simulink model "analysis_PI_ctrl_lin_uncertain_model_z"  (R2020b)
settings: Solver=FixedStepAuto  StartTime=0.0  StopTime=10.0  FixedStep=1e-3  RelTol=1e-3
values from neighbouring files (symbols this model uses):
  B = 10    [hinfCostFunc.m]    (also in hinf_analysis_z.m; hinf_cmd_lmi.m = [zeros(4,2); Sigma.B]; init_rob_synth_sim.m; muCostFunc.m = 11)
  dq0 = [0;0;0]    [hinfCostFunc.m]    (also in hinf_analysis_z.m; init_rob_synth_sim.m = [0; 0; 0]; muCostFunc.m; mu_analysis_z.m)
  Ki = 0.08    [hinfCostFunc.m]    (also in hinf_analysis_z.m; muCostFunc.m; mu_analysis_z.m; robust_synthesis.m)
  Kp = 0.015    [hinfCostFunc.m]    (also in hinf_analysis_z.m; muCostFunc.m; mu_analysis_z.m; robust_synthesis.m)
  M = 0.45    [hinfCostFunc.m]    (also in hinf_analysis_z.m; init_rob_synth_sim.m; muCostFunc.m = 0.42; mu_analysis_z.m = 0.42)
  q0 = [1.676; -4.363; 1.497]    [hinfCostFunc.m]    (also in hinf_analysis_z.m; init_rob_synth_sim.m; muCostFunc.m; mu_analysis_z.m)
  Sigma = minreal(Sigma, [], false)    [hinfCostFunc.m]    (also in hinf_analysis_z.m = youbot_lin_model_ss_z; hinf_cmd_lmi.m = youbot_lin_model_ss_z; muCostFunc.m; mu_analysis_z.m = youbot_lin_model_ss_z)
  tau_m = 1/(10*2*pi)    (= 0.0159154943092)    [hinfCostFunc.m]    (also in hinf_analysis_z.m; init_rob_synth_sim.m; muCostFunc.m; mu_analysis_z.m)
libraries: RCTblocks x1
settings Model: Creator=Fortineau_Vin  LastModifiedBy=Fortineau_Vin

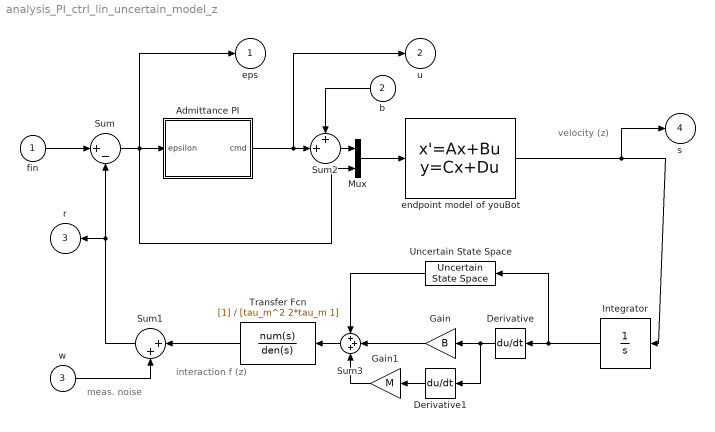
== system analysis_PI_ctrl_lin_uncertain_model_z ==
  note: velocity (z)
  note: meas. noise
  note: interaction f (z)
  fin : Inport  PortDimensions=1
  b : Inport  Port=2  PortDimensions=1
  w : Inport  Port=3  PortDimensions=1
  Admittance PI : Subsystem
  Derivative : Derivative
  Derivative1 : Derivative
  Gain : Gain  Gain=B
  Gain1 : Gain  Gain=M
  Integrator : Integrator
  Mux : Mux  Inputs=2
  Sum : Sum  Inputs=|+-
  Sum1 : Sum  Inputs=|++
  Sum2 : Sum  Inputs=++|
  Sum3 : Sum  Inputs=+++
  Transfer Fcn : TransferFcn  Denominator=[tau_m^2 2*tau_m 1]
  Uncertain State Space : RCTblocks/Uncertain State Space  Tag=USS  USystem=K  UValue=[]  X0=[]  uX0=[]
      settings: SourceProductBaseCode=RC
  endpoint model of youBot : StateSpace  A=Sigma.A  B=Sigma.B  C=Sigma.C  D=Sigma.D  InitialCondition=[q0;dq0]
  eps : Outport  PortDimensions=1
  u : Outport  Port=2  PortDimensions=1
  r : Outport  Port=3  PortDimensions=1
  s : Outport  Port=4  PortDimensions=1
  wires:
  Mux/1 -> endpoint model of youBot/1
  Admittance PI/1(cmd) -> Sum2/2, u/1
  Sum/1 -> Mux/2, eps/1, Admittance PI/1(epsilon)
  Sum2/1 -> Mux/1
  b/1 -> Sum2/1
  Sum1/1 -> Sum/2, r/1
  fin/1 -> Sum/1
  w/1 -> Sum1/2
  endpoint model of youBot/1 -> s/1, Integrator/1
  Integrator/1 -> Derivative/1, Uncertain State Space/1
  Derivative/1 -> Derivative1/1, Gain/1
  Derivative1/1 -> Gain1/1
  Gain/1 -> Sum3/2
  Gain1/1 -> Sum3/3
  Uncertain State Space/1 -> Sum3/1
  Sum3/1 -> Transfer Fcn/1
  Transfer Fcn/1 -> Sum1/1

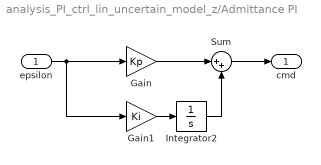
== system analysis_PI_ctrl_lin_uncertain_model_z/Admittance PI ==
  epsilon : Inport
  Gain : Gain  Gain=Kp
  Gain1 : Gain  Gain=Ki
  Integrator2 : Integrator
  Sum : Sum  Inputs=|++
  cmd : Outport  VectorParamsAs1DForOutWhenUnconnected=off
  wires:
  Integrator2/1 -> Sum/2
  Gain/1 -> Sum/1
  Gain1/1 -> Integrator2/1
  epsilon/1 -> Gain/1, Gain1/1
  Sum/1 -> cmd/1
